simulink model "EVrange"  (R2024a)
settings: Solver=FixedStepAuto  StartTime=0.0  StopTime=2000  FixedStep=1  RelTol=1e-3
libraries: simulink x4
settings Model: Creator=kaguy  LastModifiedBy=kaguy

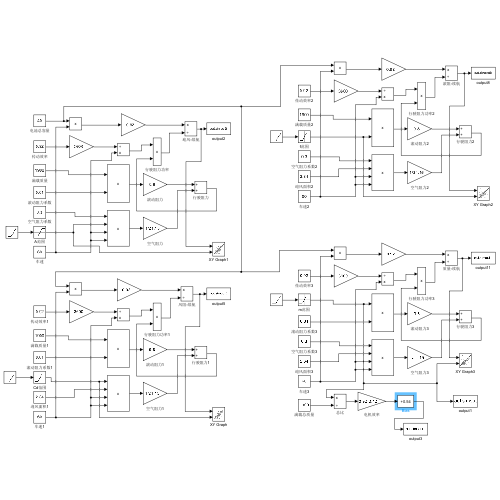
[thumbnail: Simulink's stored preview of the top-level diagram]
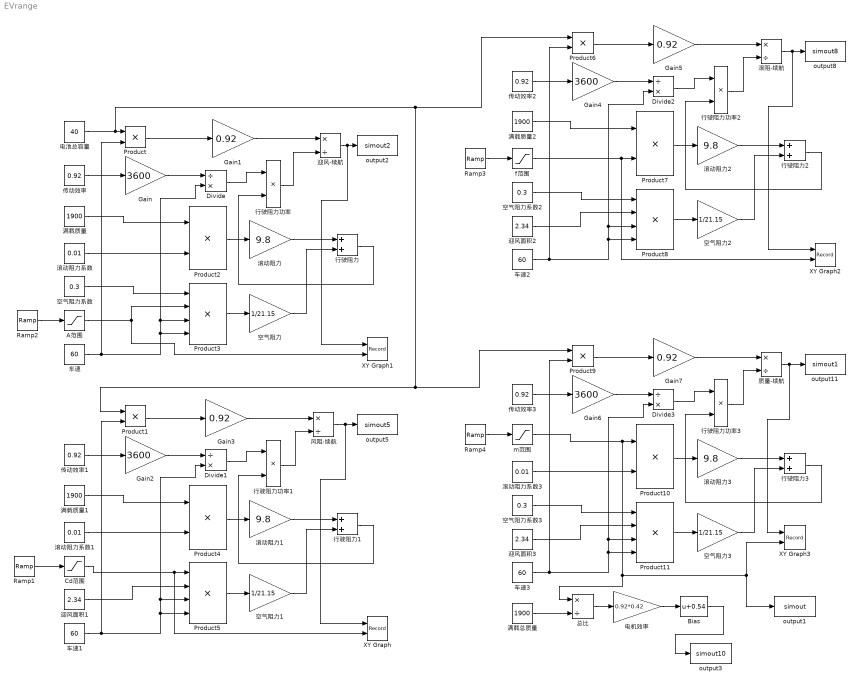
== system EVrange ==
  A范围 : Saturate  UpperLimit=4  LowerLimit=1.5
  Bias : Bias  Bias=0.54  SaturateOnIntegerOverflow=off
  Cd范围 : Saturate  UpperLimit=0.45  LowerLimit=0.25
  Divide{,1..3} (4 alike) : Product  Inputs=/*
  Gain{,2,4,6} (4 alike) : Gain  Gain=3600
  Gain{1,3,5,7} (4 alike) : Gain  Gain=0.92
  Product{,1..2,4,6..7,9..10} (8 alike) : Product
  Product{3,5,8,11} (4 alike) : Product  Inputs=4
  Ramp1 : simulink/Sources/Ramp  slope=0.001  start=0  InitialOutput=0
  Ramp2 : simulink/Sources/Ramp  slope=0.01  start=0  InitialOutput=0
  Ramp3 : simulink/Sources/Ramp  slope=0.00001  start=0  InitialOutput=0
  Ramp4 : simulink/Sources/Ramp  slope=1  start=0  InitialOutput=0
  XY Graph : Record  FileSettingsInternal="{\"entries\":[{\"content\":{\"excelSettings\":{\"content\":{},\"type\":\"Streamout.ExcelSettings\"}},\"type\":\"Streamout.FileSettingStorage\",\"uuid\":\"\"}],\"packageUris\":[\"http:\\/\\/schema.mathworks.com\\/mf0\\/streamout_blocks\\/R2020a\"],\"version\":\"1.0\"}"  Layout=[1 1]  SignalsInternal="{\"entries\":[{\"content\":{\"signals\":[{\"content\":{\"blockPath\":[],\"dimensions\":[1],\"domain\":\"\",\"lineColor\":\"#edb120\",\"lineWidth\":2,\"plots\":[ 1 ],\"port\":1,\"sid\":[\"\"],\"signalID\":1,\"signalName\":\"风阻-续航\"},\"type\":\"RecordBlkView.Signal\",\"uuid\":\"\"},{\"content\":{\"blockPath\":[],\"dimensions\":[1],\"domain\":\"\",\"lineColor\":\"#7e2f8e\",\"lineWidth\":2,\"plots\":[ 1 ],\"port\":2,\"sid\":[\"\"],\"signalID\":2,\"signalName\":\"Cd范围\"},\"type\":\"RecordBlkView.Signal\",\"uuid\":\"\"}]},\"type\":\"RecordBlkView.InputSignals\",\"uuid\":\"\"}],\"packageUris\":[\"http:\\/\\/schema.mathworks.com\\/mf0\\/streamout_blocks\\/R2020a\"],\"version\":\"1.0\"}"  VisualizationBindings="{\"xyplotplugin\":{\"info\":[{\"series\":[{\"bindingParametersList\":[{\"parameter\":\"X-Axis\",\"signalID\":2,\"signalName\":\"Cd范围\"},{\"parameter\":\"Y-Axis\",\"signalID\":1,\"signalName\":\"风阻-续航\"}],\"seriesID\":0}],\"subplotID\":1}]}}"  CompatibilityTag=XY  st=-1
  XY Graph1 : Record  FileSettingsInternal="{\"entries\":[{\"content\":{\"excelSettings\":{\"content\":{},\"type\":\"Streamout.ExcelSettings\"}},\"type\":\"Streamout.FileSettingStorage\",\"uuid\":\"\"}],\"packageUris\":[\"http:\\/\\/schema.mathworks.com\\/mf0\\/streamout_blocks\\/R2020a\"],\"version\":\"1.0\"}"  Layout=[1 1]  SignalsInternal="{\"entries\":[{\"content\":{\"signals\":[{\"content\":{\"blockPath\":[],\"dimensions\":[1],\"domain\":\"\",\"lineColor\":\"#7e2f8e\",\"lineWidth\":2,\"plots\":[ 1 ],\"port\":1,\"sid\":[\"\"],\"signalID\":1,\"signalName\":\"迎风-续航\"},\"type\":\"RecordBlkView.Signal\",\"uuid\":\"\"},{\"content\":{\"blockPath\":[],\"dimensions\":[1],\"domain\":\"\",\"lineColor\":\"#77ac30\",\"lineWidth\":2,\"plots\":[ 1 ],\"port\":2,\"sid\":[\"\"],\"signalID\":2,\"signalName\":\"A范围\"},\"type\":\"RecordBlkView.Signal\",\"uuid\":\"\"}]},\"type\":\"RecordBlkView.InputSignals\",\"uuid\":\"\"}],\"packageUris\":[\"http:\\/\\/schema.mathworks.com\\/mf0\\/streamout_blocks\\/R2020a\"],\"version\":\"1.0\"}"  VisualizationBindings="{\"xyplotplugin\":{\"info\":[{\"series\":[],\"subplotID\":1}]}}"  CompatibilityTag=XY  st=-1
  XY Graph2 : Record  FileSettingsInternal="{\"entries\":[{\"content\":{\"excelSettings\":{\"content\":{},\"type\":\"Streamout.ExcelSettings\"}},\"type\":\"Streamout.FileSettingStorage\",\"uuid\":\"\"}],\"packageUris\":[\"http:\\/\\/schema.mathworks.com\\/mf0\\/streamout_blocks\\/R2020a\"],\"version\":\"1.0\"}"  Layout=[1 1]  SignalsInternal="{\"entries\":[{\"content\":{\"signals\":[{\"content\":{\"blockPath\":[],\"dimensions\":[1],\"domain\":\"\",\"lineColor\":\"#4dbeee\",\"lineWidth\":2,\"port\":1,\"sid\":[\"\"],\"signalID\":1,\"signalName\":\"滚阻-续航\"},\"type\":\"RecordBlkView.Signal\",\"uuid\":\"\"},{\"content\":{\"blockPath\":[],\"dimensions\":[1],\"domain\":\"\",\"lineColor\":\"#a2142f\",\"lineWidth\":2,\"port\":2,\"sid\":[\"\"],\"signalID\":2,\"signalName\":\"f范围\"},\"type\":\"RecordBlkView.Signal\",\"uuid\":\"\"}]},\"type\":\"RecordBlkView.InputSignals\",\"uuid\":\"\"}],\"packageUris\":[\"http:\\/\\/schema.mathworks.com\\/mf0\\/streamout_blocks\\/R2020a\"],\"version\":\"1.0\"}"  VisualizationBindings="{\"xyplotplugin\":{\"info\":[{\"series\":[],\"subplotID\":1}]}}"  CompatibilityTag=XY  st=-1
  XY Graph3 : Record  FileSettingsInternal="{\"entries\":[{\"content\":{\"excelSettings\":{\"content\":{},\"type\":\"Streamout.ExcelSettings\"}},\"type\":\"Streamout.FileSettingStorage\",\"uuid\":\"\"}],\"packageUris\":[\"http:\\/\\/schema.mathworks.com\\/mf0\\/streamout_blocks\\/R2020a\"],\"version\":\"1.0\"}"  Layout=[1 1]  SignalsInternal="{\"entries\":[{\"content\":{\"signals\":[{\"content\":{\"blockPath\":[],\"dimensions\":[1],\"domain\":\"\",\"lineColor\":\"#ff6929\",\"lineWidth\":2,\"port\":1,\"sid\":[\"\"],\"signalID\":1,\"signalName\":\"质量-续航\"},\"type\":\"RecordBlkView.Signal\",\"uuid\":\"\"},{\"content\":{\"blockPath\":[],\"dimensions\":[1],\"domain\":\"\",\"lineColor\":\"#22b573\",\"lineWidth\":2,\"port\":2,\"sid\":[\"\"],\"signalID\":2,\"signalName\":\"m范围\"},\"type\":\"RecordBlkView.Signal\",\"uuid\":\"\"}]},\"type\":\"RecordBlkView.InputSignals\",\"uuid\":\"\"}],\"packageUris\":[\"http:\\/\\/schema.mathworks.com\\/mf0\\/streamout_blocks\\/R2020a\"],\"version\":\"1.0\"}"  VisualizationBindings="{\"xyplotplugin\":{\"info\":[{\"series\":[],\"subplotID\":1}]}}"  CompatibilityTag=XY  st=-1
  f范围 : Saturate  UpperLimit=0.018  LowerLimit=0.008
  m范围 : Saturate  UpperLimit=1900  LowerLimit=1400
  output1 : ToWorkspace  VariableName=simout  SaveFormat=Timeseries  SampleTime=-1
  output11 : ToWorkspace  VariableName=simout1  SaveFormat=Timeseries  SampleTime=-1
  output2 : ToWorkspace  VariableName=simout2  SaveFormat=Timeseries  SampleTime=-1
  output3 : ToWorkspace  VariableName=simout10  SaveFormat=Timeseries  SampleTime=-1
  output5 : ToWorkspace  VariableName=simout5  SaveFormat=Timeseries  SampleTime=-1
  output8 : ToWorkspace  VariableName=simout8  SaveFormat=Timeseries  SampleTime=-1
  传动效率{,1..3} (4 alike) : Constant  Value=0.92
  总比 : Product  Inputs=*/
  滚动阻力{,1..3} (4 alike) : Gain  Gain=9.8
  滚动阻力系数 : Constant  Value=0.01
  滚动阻力系数1 : Constant  Value=0.01
  滚动阻力系数3 : Constant  Value=0.01
  滚阻-续航 : Product  Inputs=*/
  满载总质量 : Constant  Value=1900
  满载质量 : Constant  Value=1900
  满载质量1 : Constant  Value=1900
  满载质量2 : Constant  Value=1900
  电机效率 : Gain  Gain=0.92*0.42
  电池总容量 : Constant  Value=40
  空气阻力{,1..3} (4 alike) : Gain  Gain=1/21.15
  空气阻力系数 : Constant  Value=0.3
  空气阻力系数2 : Constant  Value=0.3
  空气阻力系数3 : Constant  Value=0.3
  行驶阻力{,1..3} (4 alike) : Sum
  行驶阻力功率{,1..3} (4 alike) : Product
  质量-续航 : Product  Inputs=*/
  车速{,1..3} (4 alike) : Constant  Value=60
  迎风-续航 : Product  Inputs=*/
  迎风面积1 : Constant  Value=2.34
  迎风面积2 : Constant  Value=2.34
  迎风面积3 : Constant  Value=2.34
  风阻-续航 : Product  Inputs=*/
  wires:
  满载质量/1 -> Product2/1
  空气阻力/1 -> 行驶阻力/2
  滚动阻力/1 -> 行驶阻力/1
  Product2/1 -> 滚动阻力/1
  A范围/1 -> XY Graph1/2, Product3/2
  滚动阻力系数/1 -> Product2/2
  行驶阻力/1 -> 行驶阻力功率/2
  空气阻力系数/1 -> Product3/1
  Product3/1 -> 空气阻力/1
  Ramp2/1 -> A范围/1
  Ramp1/1 -> Cd范围/1
  Ramp3/1 -> f范围/1
  Ramp4/1 -> m范围/1
  车速/1 -> Product/2, Product3/4, Divide/2, Product3/3
  传动效率/1 -> Gain/1
  Gain/1 -> Divide/1
  行驶阻力功率/1 -> 迎风-续航/2
  Divide/1 -> 行驶阻力功率/1
  Product/1 -> Gain1/1
  Gain1/1 -> 迎风-续航/1
  迎风-续航/1 -> XY Graph1/1, output2/1
  车速1/1 -> Product1/2, Product5/4, Divide1/2, Product5/3
  风阻-续航/1 -> XY Graph/1, output5/1
  Gain3/1 -> 风阻-续航/1
  行驶阻力1/1 -> 行驶阻力功率1/2
  滚动阻力系数1/1 -> Product4/2
  Cd范围/1 -> XY Graph/2, Product5/1
  满载质量1/1 -> Product4/1
  迎风面积1/1 -> Product5/2
  空气阻力1/1 -> 行驶阻力1/2
  行驶阻力功率1/1 -> 风阻-续航/2
  Divide1/1 -> 行驶阻力功率1/1
  传动效率1/1 -> Gain2/1
  Product1/1 -> Gain3/1
  滚动阻力1/1 -> 行驶阻力1/1
  Product4/1 -> 滚动阻力1/1
  Product5/1 -> 空气阻力1/1
  Gain2/1 -> Divide1/1
  车速2/1 -> Product6/2, Product8/4, Divide2/2, Product8/3
  滚阻-续航/1 -> XY Graph2/1, output8/1
  Gain5/1 -> 滚阻-续航/1
  行驶阻力2/1 -> 行驶阻力功率2/2
  f范围/1 -> XY Graph2/2, Product7/2
  空气阻力系数2/1 -> Product8/1
  满载质量2/1 -> Product7/1
  迎风面积2/1 -> Product8/2
  空气阻力2/1 -> 行驶阻力2/2
  行驶阻力功率2/1 -> 滚阻-续航/2
  Divide2/1 -> 行驶阻力功率2/1
  传动效率2/1 -> Gain4/1
  Product6/1 -> Gain5/1
  滚动阻力2/1 -> 行驶阻力2/1
  Product7/1 -> 滚动阻力2/1
  Product8/1 -> 空气阻力2/1
  Gain4/1 -> Divide2/1
  车速3/1 -> Product9/2, Product11/4, Divide3/2, Product11/3
  质量-续航/1 -> XY Graph3/1, output11/1
  Gain7/1 -> 质量-续航/1
  行驶阻力3/1 -> 行驶阻力功率3/2
  滚动阻力系数3/1 -> Product10/2
  空气阻力系数3/1 -> Product11/1
  m范围/1 -> 总比/1, output1/1, XY Graph3/2, Product10/1
  迎风面积3/1 -> Product11/2
  空气阻力3/1 -> 行驶阻力3/2
  行驶阻力功率3/1 -> 质量-续航/2
  Divide3/1 -> 行驶阻力功率3/1
  传动效率3/1 -> Gain6/1
  电池总容量/1 -> Product9/1, Product1/1, Product6/1, Product/1
  Product9/1 -> Gain7/1
  滚动阻力3/1 -> 行驶阻力3/1
  Product10/1 -> 滚动阻力3/1
  Product11/1 -> 空气阻力3/1
  Gain6/1 -> Divide3/1
  满载总质量/1 -> 总比/2
  总比/1 -> 电机效率/1
  电机效率/1 -> Bias/1
  Bias/1 -> output3/1
